simulink model "UnicyleModel"  (R2021a)
settings: Solver=VariableStepAuto  StartTime=0.0  StopTime=50.0  RelTol=1e-3
libraries: simulink x1
settings Model: Creator=haluk  LastModifiedBy=haluk

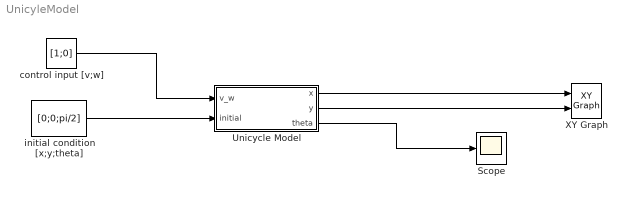
== system UnicyleModel ==
  Scope : Scope
  Unicycle Model : Subsystem
  XY Graph : simulink/Sinks/XY Graph  xmin=-10  xmax=10  ymin=-10  ymax=10  st=-1
  control input [v;w] : Constant  Value=[1;0]
  initial condition [x;y;theta] : Constant  Value=[0;0;pi/2]
  wires:
  control input [v;w]/1 -> Unicycle Model/1(v_w)
  initial condition [x;y;theta]/1 -> Unicycle Model/2(initial)
  Unicycle Model/1(x) -> XY Graph/1
  Unicycle Model/2(y) -> XY Graph/2
  Unicycle Model/3(theta) -> Scope/1

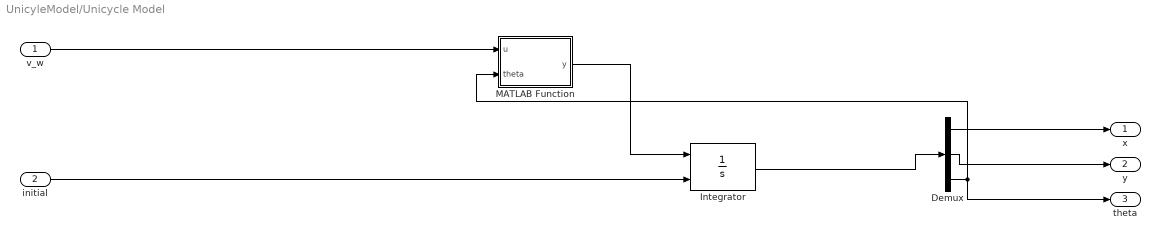
== system UnicyleModel/Unicycle Model ==
  v_w : Inport
  initial : Inport  Port=2
  Demux : Demux  Outputs=3
  Integrator : Integrator  InitialConditionSource=external
  MATLAB Function : MATLAB Function  TreatAsAtomicUnit=on
  x : Outport
  y : Outport  Port=2
  theta : Outport  Port=3
  wires:
  MATLAB Function/1(y) -> Integrator/1
  Demux/3 -> theta/1, MATLAB Function/2(theta)
  Integrator/1 -> Demux/1
  Demux/1 -> x/1
  initial/1 -> Integrator/2
  v_w/1 -> MATLAB Function/1(u)
  Demux/2 -> y/1

== matlab function UnicyleModel/Unicycle Model/MATLAB Function ==
  data: u input; y output; theta input
function y = fcn(u, theta)


v = u(1);
w = u(2);

y = [v*cos(theta); v*sin(theta); w];
